simulink model "untitled"  (R2020b)
settings: Solver=VariableStepAuto  StartTime=0.0  StopTime=10.0  RelTol=1e-3
settings Model: Creator=Administrator  LastModifiedBy=Administrator

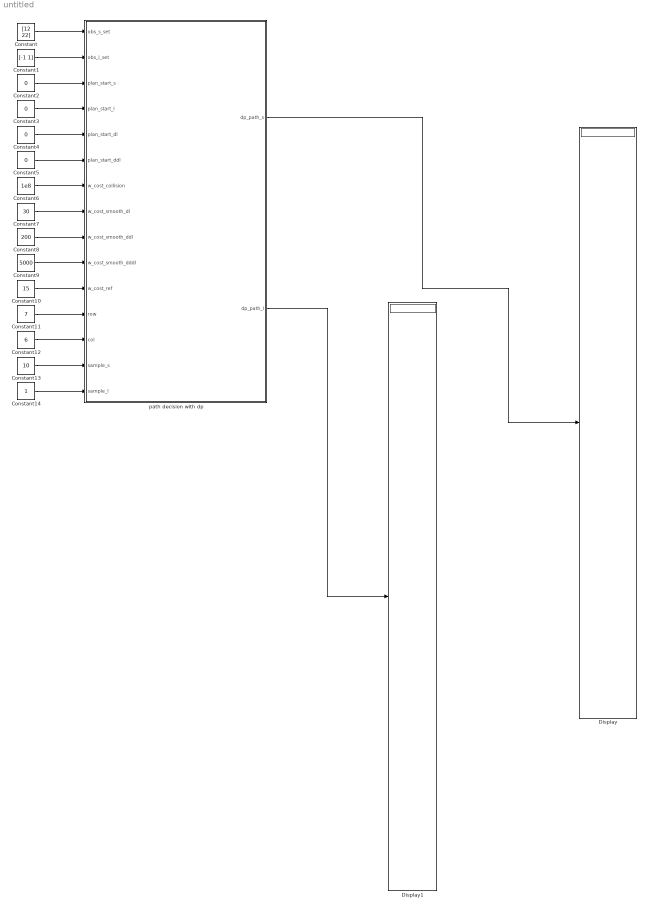
== system untitled ==
  Constant : Constant  Value=[12 22]
  Constant1 : Constant  Value=[-1 1]
  Constant10 : Constant  Value=15
  Constant11 : Constant  Value=7
  Constant12 : Constant  Value=6
  Constant13 : Constant  Value=10
  Constant14 : Constant
  Constant{2..5} (4 alike) : Constant  Value=0
  Constant6 : Constant  Value=1e8
  Constant7 : Constant  Value=30
  Constant8 : Constant  Value=200
  Constant9 : Constant  Value=5000
  Display : Display
  Display1 : Display
  path decision with dp : MATLAB Function  TreatAsAtomicUnit=on
  wires:
  Constant/1 -> path decision with dp/1(obs_s_set)
  Constant1/1 -> path decision with dp/2(obs_l_set)
  Constant2/1 -> path decision with dp/3(plan_start_s)
  Constant3/1 -> path decision with dp/4(plan_start_l)
  Constant4/1 -> path decision with dp/5(plan_start_dl)
  Constant5/1 -> path decision with dp/6(plan_start_ddl)
  Constant6/1 -> path decision with dp/7(w_cost_collision)
  Constant7/1 -> path decision with dp/8(w_cost_smooth_dl)
  Constant8/1 -> path decision with dp/9(w_cost_smooth_ddl)
  Constant9/1 -> path decision with dp/10(w_cost_smooth_dddl)
  Constant10/1 -> path decision with dp/11(w_cost_ref)
  Constant11/1 -> path decision with dp/12(row)
  Constant12/1 -> path decision with dp/13(col)
  Constant13/1 -> path decision with dp/14(sample_s)
  Constant14/1 -> path decision with dp/15(sample_l)
  path decision with dp/1(dp_path_s) -> Display/1
  path decision with dp/2(dp_path_l) -> Display1/1

== matlab function untitled/path decision with dp ==
  data: obs_s_set input; dp_path_s output; obs_l_set input; plan_start_s input; plan_start_l input; plan_start_dl input; plan_start_ddl input; w_cost_collision input; w_cost_smooth_dl input; w_cost_smooth_ddl input; w_cost_smooth_dddl input; w_cost_ref input; dp_path_l output; row input; col input; sample_s input; sample_l input
function [dp_path_s,dp_path_l] = fcn(obs_s_set,obs_l_set,plan_start_s,plan_start_l,plan_start_dl,plan_start_ddl,...
    w_cost_collision,w_cost_smooth_dl,w_cost_smooth_ddl,w_cost_smooth_dddl,w_cost_ref,row,col,sample_s,sample_l)
% 该函数为路径决策算法：动态规划的主函数
% 输入: obs_s_set,obs_l_set 筛选后的障碍物sl
%     plan_start_s,plan_start_l,plan_start_dl,plan_start_ddl 规划起点信息
%     w_cost_obs,w_cost_smooth_dl,w_cost_smooth_ddl,w_cost_smooth_dddl,w_cost_ref动态规划的代价权重
%     row col 动态规划的行和列

%   从起点到行为i 列为j的采样点所花费的最短代价记为node_cost(i,j)
    node_cost = ones(row,col)*inf;
%   行为i，列为j的采样点的前一层中，最小代价的采样点的行号记为pre_node(i,j)
    pre_node_index = zeros(row,col);
    %初始化
    for i = 1:row
        node_cost(i,1) = CalcStartCost(plan_start_s,plan_start_l,plan_start_dl,plan_start_ddl,i,...
            w_cost_collision,w_cost_smooth_dl,w_cost_smooth_ddl,w_cost_smooth_dddl,w_cost_ref,obs_s_set,obs_l_set,sample_s,sample_l,row);
    end
    %动态规划主函数
    for j = 2:col
        for i = 1:row
            for k = 1:row
                start_s = (j-1)*sample_s + plan_start_s;
                cost_neighbour = CalcNeighbourCost(k,i,w_cost_collision,w_cost_smooth_dl,...
                    w_cost_smooth_ddl,w_cost_smooth_dddl,w_cost_ref,obs_s_set,obs_l_set,start_s,sample_s,sample_l,row);
                cost_temp = cost_neighbour + node_cost(k,j-1);
                if cost_temp <= node_cost(i,j)
                    node_cost(i,j) = cost_temp;
                    pre_node_index(i,j) = k;
                end
            end
        end
    end
    %找到矩阵最末端的一列中，代价函数最小的，记代价最小的行号为index
    index = 0;
    min_cost = inf;
    for i = 1:col
        if  node_cost(i,end) < min_cost
            min_cost = node_cost(i,end);
            index = i;
        end
    end
    %最短路径初始化
    index_list = zeros(col,1);
    %从后往前逆推
    cur_index = index;
    for i = 1:col    
        pre_index = pre_node_index(cur_index,end - i + 1);
        index_list(col - i + 1) = cur_index;
        cur_index = pre_index;
    end
    %index_list就是最短路径点的行的编号
    %输出初始化
    dp_path_s = zeros(120,1);
    dp_path_l = zeros(120,1);
    for i = 1:length(index_list)
        if i == 1
            start_l = plan_start_l;
            start_dl = plan_start_dl;
            start_ddl = plan_start_ddl;
            end_l = ((row + 1)/2 - index_list(i)) * sample_l;
            end_dl = 0;
            end_ddl = 0;
            ds = sample_s;
            s = zeros(20,1);
            for j = 1:20
                s(j) = j*ds/20;
            end
            coeff = CalcQuinticCoffient(start_l,start_dl,start_ddl,end_l,end_dl,end_ddl,ds);
            l = ones(20,1)*coeff(1) + s*coeff(2) + s.^2*coeff(3) + s.^3*coeff(4) + s.^4*coeff(5) + s.^5*coeff(6);
            s_real = s + ones(20,1)*plan_start_s;
            l_real = l;
            dp_path_s(20*i - 19:20*i) = s_real;
            dp_path_l(20*i - 19:20*i) = l_real;
        else
            start_l = 0;
            start_dl = 0;
            start_ddl = 0;
            end_l = (index_list(i - 1) - index_list(i)) * sample_l;
            end_dl = 0;
            end_ddl = 0;
            ds = sample_s;
            s = zeros(20,1);
            for j = 1:20
                s(j) = j*ds/20;
            end
            coeff = CalcQuinticCoffient(start_l,start_dl,start_ddl,end_l,end_dl,end_ddl,ds);
            l = ones(20,1)*coeff(1) + s*coeff(2) + s.^2*coeff(3) + s.^3*coeff(4) + s.^4*coeff(5) + s.^5*coeff(6);
            s_real = s + ones(20,1)*((i-1)*sample_s + plan_start_s);
            l_real = l + ones(20,1)*sample_l*((row + 1)/2 - index_list(i - 1)); 
            dp_path_s(20*i - 19:20*i) = s_real;
            dp_path_l(20*i - 19:20*i) = l_real;
            
        end
    end
    
    
  
    
end

function cost = CalcNeighbourCost(pre_node_row,cur_node_row,w_cost_collision,w_cost_smooth_dl,...
    w_cost_smooth_ddl,w_cost_smooth_dddl,w_cost_ref,obs_s_set,obs_l_set,start_s,sample_s,sample_l,row)
    %该函数计算相邻两列节点的cost
    start_l = 0;
    start_dl = 0;
    start_ddl = 0;
    end_l = (pre_node_row - cur_node_row)*sample_l;
    end_dl = 0;
    end_ddl = 0;
    ds = sample_s;
    %计算系数
    coeff = CalcQuinticCoffient(start_l,start_dl,start_ddl,end_l,end_dl,end_ddl,ds);
    %取10个点
    s = zeros(10,1);
    for i = 1:10
        s(i) = i*ds/10;
    end
    l = ones(10,1)*coeff(1) + s*coeff(2) + s.^2*coeff(3) + s.^3*coeff(4) + s.^4*coeff(5) + s.^5*coeff(6);
    dl = ones(10,1)*coeff(2) + 2*s*coeff(3) + 3*s.^2*coeff(4) + 4*s.^3*coeff(5) + 5*s.^4*coeff(6);
    ddl = 2*ones(10,1)*coeff(3) + 6*s*coeff(4) + 12*s.^2*coeff(5) + 20*s.^3*coeff(6);
    dddl = 6*ones(10,1)*coeff(4) + 24*s*coeff(5) + 60*s.^2*coeff(6);
    s_real = s + ones(10,1)*start_s;
    l_real = l + ones(10,1)*sample_l*((row + 1)/2 - pre_node_row); 
    cost_smooth = w_cost_smooth_dl * (dl' * dl) + w_cost_smooth_ddl * (ddl' * ddl) + w_cost_smooth_dddl * (dddl' * dddl);
    cost_ref = w_cost_ref * (l_real' * l_real);
    cost_collision = 0;
    for i = 1:length(obs_s_set)
        if isnan(obs_s_set(i))
            break;
        end
        dlon = ones(10,1)*obs_s_set(i) - s_real;
        dlat = ones(10,1)*obs_l_set(i) - l_real;
        square_d = dlon.^2 + dlat.^2;
        cost_temp = CalcObsCost(w_cost_collision,square_d);
        cost_collision = cost_collision + cost_temp;
    end
    cost = cost_smooth + cost_ref + cost_collision;
end


function cost = CalcStartCost(s_begin,l,dl,ddl,cur_row,w_cost_collision,w_cost_smooth_dl,...
    w_cost_smooth_ddl,w_cost_smooth_dddl,w_cost_ref,obs_s_set,obs_l_set,sample_s,sample_l,row)
    %该函数计算起点到第一层的cost
    start_l = l;
    start_dl = dl;
    start_ddl = ddl;
    end_l = ((row + 1)/2 - cur_row)*sample_l;
    end_dl = 0;
    end_ddl = 0;
    ds = sample_s;
    %计算系数
    coeff = CalcQuinticCoffient(start_l,start_dl,start_ddl,end_l,end_dl,end_ddl,ds);
    %取10个点
    s = zeros(10,1);
    for i = 1:10
        s(i) = i*ds/10;
    end
    
    l = ones(10,1)*coeff(1) + s*coeff(2) + s.^2*coeff(3) + s.^3*coeff(4) + s.^4*coeff(5) + s.^5*coeff(6);
    dl = ones(10,1)*coeff(2) + 2*s*coeff(3) + 3*s.^2*coeff(4) + 4*s.^3*coeff(5) + 5*s.^4*coeff(6);
    ddl = 2*ones(10,1)*coeff(3) + 6*s*coeff(4) + 12*s.^2*coeff(5) + 20*s.^3*coeff(6);
    dddl = 6*ones(10,1)*coeff(4) + 24*s*coeff(5) + 60*s.^2*coeff(6);
    s_real = s + ones(10,1)*s_begin;
    l_real = l; 
    cost_smooth = w_cost_smooth_dl * (dl' * dl) + w_cost_smooth_ddl * (ddl' * ddl) + w_cost_smooth_dddl * (dddl' * dddl);
    cost_ref = w_cost_ref * (l_real'*l_real);
    cost_collision = 0;
    for i = 1:length(obs_s_set)
        if isnan(obs_s_set(i))
            break;
        end
        dlon = ones(10,1)*obs_s_set(i) - s_real;
        dlat = ones(10,1)*obs_l_set(i) - l_real;
        square_d = dlon.^2 + dlat.^2;
        cost_temp = CalcObsCost(w_cost_collision,square_d);
        cost_collision = cost_collision + cost_temp;
    end
    cost = cost_smooth + cost_ref + cost_collision;
end

function y = CalcQuinticCoffient(start_l,start_dl,start_ddl,end_l,end_dl,end_ddl,ds)
    %该函数计算start_s为0，end_s为ds的五次多项式的系数
    a0 = start_l;
    a1 = start_dl;
    a2 = start_ddl/2;
    A = [ds^3,ds^4,ds^5;
        3*ds^2,4*ds^3,5*ds^4;
        6*ds,12*ds^2,20*ds^3];
    B = [end_l - start_l - start_dl*ds - start_ddl*ds^2/2;
        end_dl - start_dl - start_ddl*ds;
        end_ddl - start_ddl];
    x = A\B;
    a3 = x(1);
    a4 = x(2);
    a5 = x(3);
    y = [a0,a1,a2,a3,a4,a5];
end

function obs_cost = CalcObsCost(w_cost_collision,square_d)
%该函数计算障碍物的距离代价
   cost = w_cost_collision*10.^(-1.5*square_d);
   obs_cost = sum(cost);
end
